simulink model "SMA_displacementIn_PC2"  (R2016a)
settings: Solver=ode15s  StartTime=0.0  StopTime=400  RelTol=1e-8  AbsTol=1e-8
libraries: simulink x1
settings Model: Creator=Gianluca  LastModifiedBy=Gianluca
settings DataIOCC: LimitDataPoints=on  SaveFormat=Array
settings DebuggingCC: UnderspecifiedInitializationDetection=Classic  MergeDetectMultiDrivingBlocksExec=none  SolverPrmCheckMsg=warning  StateNameClashWarn=warning
settings HardwareCC: ProdBitPerPointer=32  ProdLargestAtomicFloat=None  ProdIntDivRoundTo=Undefined  ProdEndianess=Unspecified  ProdWordSize=32  ProdHWDeviceType=32-bit Generic
settings ModelReferenceCC: PropagateSignalLabelsOutOfModel=off
settings ConfigComp: CovModelRefEnable=Off

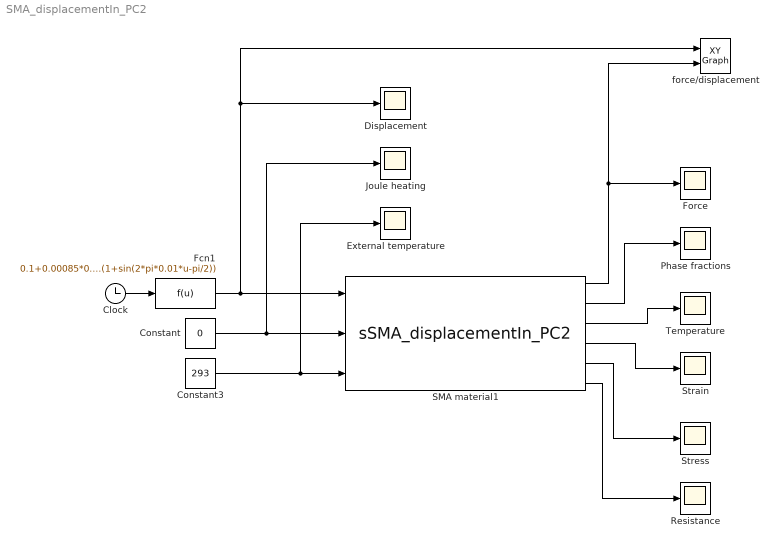
== system SMA_displacementIn_PC2 ==
  Clock : Clock
  Constant : Constant  Value=0
  Constant3 : Constant  Value=293
  Displacement : Scope
  External temperature : Scope
  Fcn1 : Fcn  Expr=0.1+0.00085*0.01*u*(1+sin(2*pi*0.01*u-pi/2))
  Force : Scope
  Joule heating : Scope
  Phase fractions : Scope
  Resistance : Scope
  SMA material1 : M-S-Function  FunctionName=sSMA_displacementIn_PC2  Parameters=params_PC2, initConds_PC2
      mask Display:
      | color('black');
      | patch(3*[-1 1 1 -1],1.1*[-1 -1 1 1],[1 1 1]);
      | patch([-1.6 -0.8],[-0.9 0.3],[0 0 0]);
      | patch([-0.8 1.2],[0.3 0.3],[0 0 0]);
      | patch([1.6 0.8],[0.9 -0.3],[0 0 0]);
      | patch([0.8 -1.2],[-0.3 -0.3],[0 0 0]);
      | disp('SMA');
      | 
      | color('blue');
      | port_label('input', 1, 'y [m]','texmode','on');
      | port_label('input', 2, 'J [W]','texmode','on');
      | port_label('input', 3, 'T_E [K]','texmode','on');
      | 
      | color('red');
      | port_label('output', 1, 'F [N]','texmode','on');
      | port_label('output', 2, 'x_+, x_-, x_A [-]','texmode','on');
      | port_label('output', 3, 'T [K]','texmode','on');
      | port_label('output', 4, '\epsilon [-]','texmode','on');
      | port_label('output', 5, '\sigma [Pa]','texmode','on');
      | port_label('output', 6, 'R [\Omega]','texmode','on');
  Strain : Scope
  Stress : Scope
  Temperature : Scope
  force/displacement : simulink/Sinks/XY Graph  xmin=0.1  xmax=0.106  ymin=0  ymax=2.5  st=-1
  wires:
  Constant/1 -> Joule heating/1, SMA material1/2
  Constant3/1 -> SMA material1/3, External temperature/1
  SMA material1/2 -> Phase fractions/1
  SMA material1/3 -> Temperature/1
  SMA material1/4 -> Strain/1
  SMA material1/5 -> Stress/1
  SMA material1/6 -> Resistance/1
  Fcn1/1 -> SMA material1/1, force/displacement/1, Displacement/1
  SMA material1/1 -> force/displacement/2, Force/1
  Clock/1 -> Fcn1/1
